simulink model "ode45alike"  (R2017a)
settings: Solver=VariableStepAuto  StartTime=0.0  StopTime=5  RelTol=1e-3
settings Model: Creator=eruffaldi  LastModifiedBy=eruffaldi

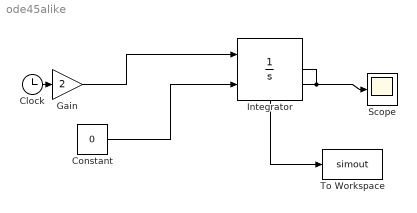
== system ode45alike ==
  Clock : Clock
  Constant : Constant  Value=0
  Gain : Gain  Gain=2
  Integrator : Integrator  InitialConditionSource=external
  Scope : Scope
  To Workspace : ToWorkspace  VariableName=simout  SaveFormat=Timeseries  SampleTime=-1
  wires:
  Clock/1 -> Gain/1
  Integrator/1 -> To Workspace/1, Scope/1
  Constant/1 -> Integrator/2
  Gain/1 -> Integrator/1
